simulink model "sinwave"  (R2014a)
settings: Solver=ode45  StartTime=0.0  StopTime=10.0  RelTol=1e-3
settings Model: Creator=naina  LastModifiedBy=naina

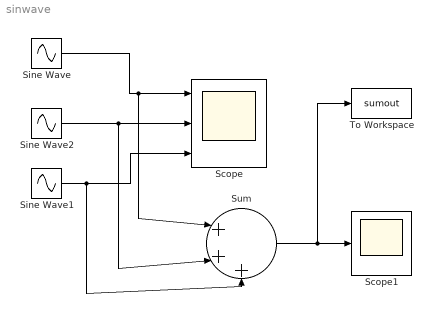
== system sinwave ==
  Scope : Scope  NumInputPorts=3
      settings: YMin=-5~-5~-5  YMax=5~5~5
  Scope1 : Scope
  Sine Wave : Sin  SampleTime=0
  Sine Wave1 : Sin  Frequency=3  SampleTime=0
  Sine Wave2 : Sin  Frequency=2  SampleTime=0
  Sum : Sum  Inputs=|+++
  To Workspace : ToWorkspace  VariableName=sumout  SaveFormat=Timeseries  SampleTime=-1
  wires:
  Sine Wave1/1 -> Sum/3, Scope/3
  Sine Wave2/1 -> Sum/2, Scope/2
  Sine Wave/1 -> Sum/1, Scope/1
  Sum/1 -> To Workspace/1, Scope1/1
